simulink model "ex4"  (R2020a)
settings: Solver=ode45  StartTime=0.0  StopTime=10.0  RelTol=1e-3  EnableMultiTasking=on
values from neighbouring files (symbols this model uses):
  A = gss.a    [ex4 .m]
  B = gss.b    [ex4 .m]
  C = gss.c    [ex4 .m]
  K = Ka(1,[1,2])    [ex4 .m]
  Kz = Ka(1,3)    [ex4 .m]
  L = lqe(A,B,C,Qn,Rn)    [ex4 .m]
settings Model: Creator=Xrisostomos  LastModifiedBy=xriso
settings DataIOCC: LimitDataPoints=on  SaveFormat=Array  ReturnWorkspaceOutputs=off
settings OptimizationCC: LifeSpan=inf
settings DebuggingCC: SFUnexpectedBacktrackingDiag=warning  SFNoUnconditionalDefaultTransitionDiag=warning  SFExecutionAtInitializationDiag=none  ArithmeticOperatorsInVariantConditions=warning
settings HardwareCC: ProdBitPerPointer=32  ProdBitPerSizeT=32  ProdBitPerPtrDiffT=32  ProdLargestAtomicFloat=None  ProdIntDivRoundTo=Undefined  ProdEndianess=Unspecified  ProdWordSize=32  ProdHWDeviceType=32-bit Generic
settings ModelReferenceCC: PropagateSignalLabelsOutOfModel=off
settings SFSimCC: SimUseLocalCustomCode=off  CustomCodeUndefinedFunction=UseInterfaceOnly
settings RTWCC: RTWUseLocalCustomCode=off
settings CodeAppCC: StateflowObjectComments=on
settings GRTTargetCC: TargetLangStandard=C89/C90 (ANSI)
settings ConfigComp: CovMetricSettings=dw  CovHtmlReporting=on  CovSaveCumulativeToWorkspaceVar=on  CovSaveSingleToWorkspaceVar=on  CovExternalEMLEnable=off

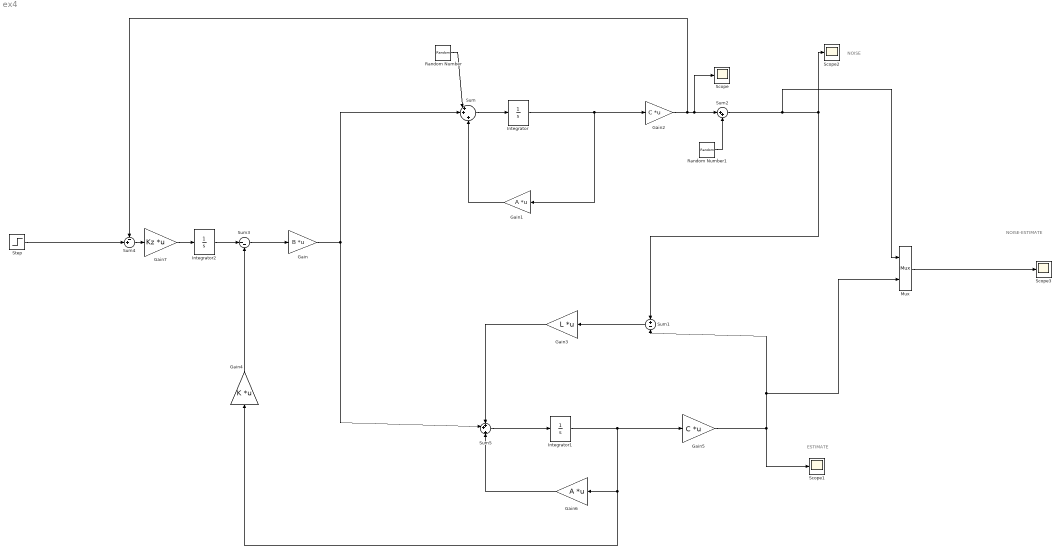
== system ex4 ==
  note: NOISE-ESTIMATE
  note: NOISE
  note: ESTIMATE
  Gain : Gain  Gain=B  Multiplication=Matrix(K*u)
  Gain1 : Gain  Gain=A  Multiplication=Matrix(K*u)
  Gain2 : Gain  Gain=C  Multiplication=Matrix(K*u)
  Gain3 : Gain  Gain=L  Multiplication=Matrix(K*u)
  Gain4 : Gain  Gain=K  Multiplication=Matrix(K*u)
  Gain5 : Gain  Gain=C  Multiplication=Matrix(K*u)
  Gain6 : Gain  Gain=A  Multiplication=Matrix(K*u)
  Gain7 : Gain  Gain=Kz  Multiplication=Matrix(K*u)
  Integrator : Integrator  InitialCondition=[1 1]
  Integrator1 : Integrator  InitialCondition=[0 0]
  Integrator2 : Integrator
  Mux : Mux  Inputs=2
  Random Number : RandomNumber  SampleTime=0.1
  Random Number1 : RandomNumber  SampleTime=0.1
  Scope{,1..3} (4 alike) : Scope
  Step : Step  SampleTime=0
  Sum : Sum  Inputs=|++|+
  Sum1 : Sum  Inputs=+|-
  Sum2 : Sum  Inputs=|++
  Sum3 : Sum  Inputs=|--
  Sum4 : Sum  Inputs=-+|
  Sum5 : Sum  Inputs=++|+
  wires:
  Gain/1 -> Sum/2, Sum5/2
  Sum/1 -> Integrator/1
  Integrator/1 -> Gain2/1, Gain1/1
  Gain1/1 -> Sum/3
  Gain3/1 -> Sum5/1
  Sum5/1 -> Integrator1/1
  Gain6/1 -> Sum5/3
  Integrator1/1 -> Gain5/1, Gain4/1, Gain6/1
  Sum1/1 -> Gain3/1
  Sum2/1 -> Sum1/1, Scope2/1, Mux/1
  Gain2/1 -> Sum4/1, Scope/1, Sum2/1
  Gain5/1 -> Sum1/2, Mux/2, Scope1/1
  Random Number/1 -> Sum/1
  Random Number1/1 -> Sum2/2
  Mux/1 -> Scope3/1
  Sum3/1 -> Gain/1
  Gain7/1 -> Integrator2/1
  Integrator2/1 -> Sum3/1
  Gain4/1 -> Sum3/2
  Sum4/1 -> Gain7/1
  Step/1 -> Sum4/2
